simulink model "Ourobouros"  (R2024a)
settings: Solver=VariableStepAuto  StartTime=0.0  StopTime=20.0  RelTol=1e-3
model workspace (MAT data in the model file):
  Tsplant = 0.001
settings Model: Creator=Marij  LastModifiedBy=Marij
settings OptimizationCC: UseDivisionForNetSlopeComputation=on

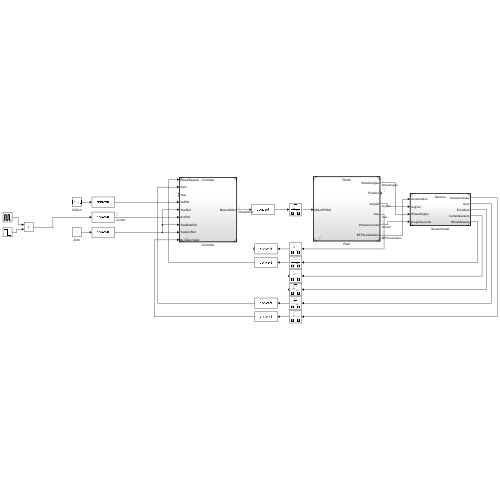
[thumbnail: Simulink's stored preview of the top-level diagram]
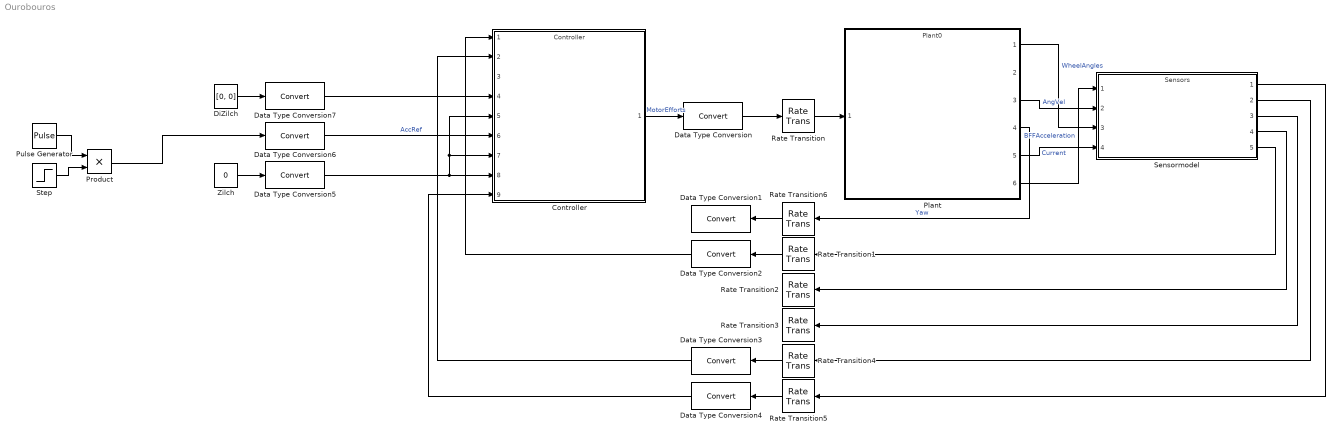
== system Ourobouros ==
  Controller : ModelReference  ModelNameDialog=Controller.slx  SimulationMode=Normal  ModelReferenceVersion=1.153
  Data Type Conversion{,1..7} (8 alike) : DataTypeConversion  SaturateOnIntegerOverflow=off  RndMeth=Floor
  DiZilch : Constant  Value=[0, 0]
  Plant : ModelReference  ModelNameDialog=Plant0.slx  SimulationMode=Normal  ModelReferenceVersion=1.26
  Product : Product
  Pulse Generator : DiscretePulseGenerator  PulseType=Time based  Amplitude=[1, 0]  Period=[10, 10]  PulseWidth=[50, 50]  PhaseDelay=[2.5, 5]  VectorParams1D=off
  Rate Transition : RateTransition  OutPortSampleTime=Tsplant
  Rate Transition{1..6} (6 alike) : RateTransition  OutPortSampleTime=1e-2
  Sensormodel : ModelReference  ModelNameDialog=Sensors.slx  SimulationMode=Normal  ModelReferenceVersion=1.6
  Step : Step  Time=5  Before=1  After=0  SampleTime=0
  Zilch : Constant  Value=0
  wires:
  Controller/1 -> Data Type Conversion/1  "MotorEfforts"
  Plant/1 -> Sensormodel/3  "WheelAngles"
  Plant/6 -> Sensormodel/1  "BFFAcceleration"
  Plant/3 -> Sensormodel/2  "AngVel"
  Plant/5 -> Sensormodel/4  "Current"
  Rate Transition/1 -> Plant/1
  Sensormodel/5 -> Rate Transition1/1
  Sensormodel/4 -> Rate Transition2/1
  Sensormodel/3 -> Rate Transition3/1
  Sensormodel/2 -> Rate Transition4/1
  Sensormodel/1 -> Rate Transition5/1
  Rate Transition1/1 -> Data Type Conversion2/1
  Rate Transition4/1 -> Data Type Conversion3/1
  Rate Transition5/1 -> Data Type Conversion4/1
  Plant/4 -> Rate Transition6/1  "Yaw"
  Rate Transition6/1 -> Data Type Conversion1/1
  Data Type Conversion/1 -> Rate Transition/1
  Data Type Conversion2/1 -> Controller/1
  Data Type Conversion3/1 -> Controller/2
  Data Type Conversion4/1 -> Controller/9
  Zilch/1 -> Data Type Conversion5/1
  DiZilch/1 -> Data Type Conversion7/1
  Data Type Conversion5/1 -> Controller/5, Controller/7, Controller/8
  Data Type Conversion6/1 -> Controller/6  "AccRef"
  Data Type Conversion7/1 -> Controller/4
  Step/1 -> Product/2
  Pulse Generator/1 -> Product/1
  Product/1 -> Data Type Conversion6/1
